simulink model "droop_model"  (R2023a)
settings: Solver=VariableStepAuto  StartTime=0.0  StopTime=6  RelTol=1e-3
values from neighbouring files (symbols this model uses):
  BESS2 =     [state_space.mat]    (also in state_space_and_controllers.mat)
  Grid =     [state_space.mat]    (also in state_space_and_controllers.mat)
  Load =     [state_space.mat]    (also in state_space_and_controllers.mat)
  PV1 =     [state_space.mat]    (also in state_space_and_controllers.mat)
  Ts = 0.0001    [cost_analysis.m]    (also in simulation_run.m)
undefined symbols (not defined in the file or in its folder): A1, A2, B1, B2, C1, C2, K1_integral, K1_proportional, K2_integral, K2_proportional
libraries: slpidlib x5, spspowerguiLib x1
settings Model: Creator=paul  LastModifiedBy=paul
settings DataIOCC: Refine=4

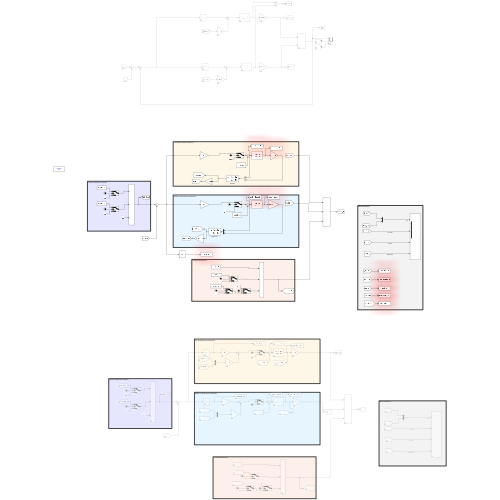
[thumbnail: Simulink's stored preview of the top-level diagram]
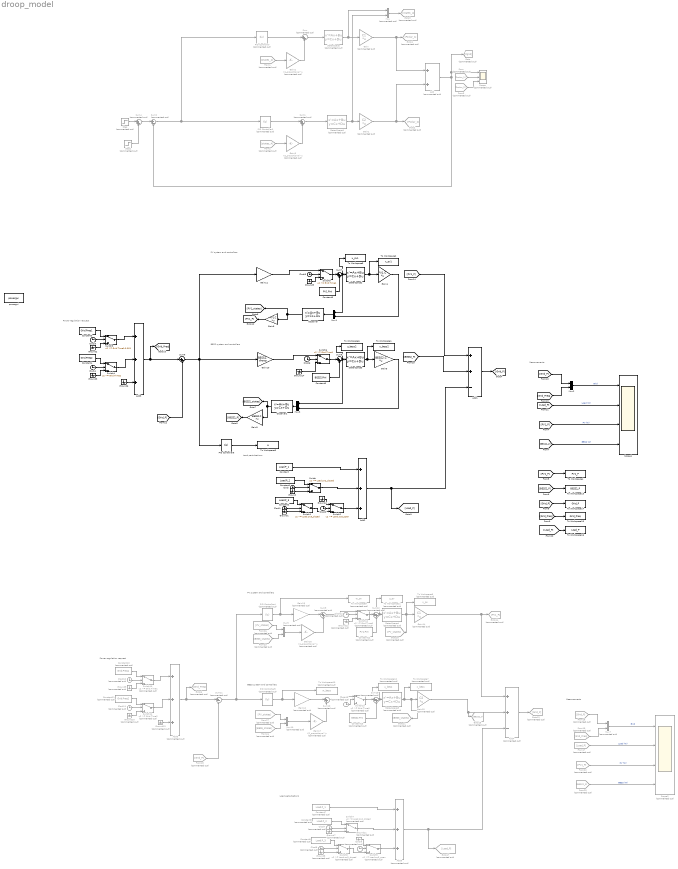
== system droop_model ==
  note: BESS system and controllers
  note: Measurements
  note: PV system and controllers
  note: Load perturbations
  note: Power regulation request
  note: BESS system and controllers
  note: Load perturbations
  note: Measurements
  note: Power regulation request
  note: PV system and controllers
  Add : Sum  Commented=on
  Add1 : Sum  Inputs=++-
  Add2 : Sum  Inputs=+++
  Add3 : Sum  Inputs=+++
  Add4 : Sum  Commented=on  Inputs=++-
  Add5 : Sum  Commented=on  Inputs=+++
  Add6 : Sum  Commented=on  Inputs=+++
  Clock{,1..6} (7 alike) : Clock
  Clock{7..13} (7 alike) : Clock  Commented=on
  Constant : Constant  Value=Load.P_1
  Constant1 : Constant  Value=Load.P_2
  Constant10 : Constant  Commented=on  Value=Grid.Preq1
  Constant11 : Constant  Commented=on  Value=Grid.Preq2
  Constant12 : Constant  Commented=on  Value=PV1.Pini
  Constant13 : Constant  Commented=on  Value=BESS2.Pini
  Constant2 : Constant  Value=Load.P_3
  Constant3 : Constant  Value=Grid.Preq1
  Constant4 : Constant  Value=Grid.Preq2
  Constant5 : Constant  Value=PV1.Pini
  Constant6 : Constant  Value=BESS2.Pini
  Constant7 : Constant  Commented=on  Value=Load.P_1
  Constant8 : Constant  Commented=on  Value=Load.P_2
  Constant9 : Constant  Commented=on  Value=Load.P_3
  From : From  Commented=on  GotoTag=Psolar_1
  From1 : From  Commented=on  GotoTag=states_4
  From16 : From  Commented=on  GotoTag=Grid_P
  From17 : From  Commented=on  GotoTag=Load_P
  From18 : From  Commented=on  GotoTag=Grid_P
  From19 : From  Commented=on  GotoTag=Grid_Preq
  From2 : From  Commented=on  GotoTag=states_4
  From22 : From  Commented=on  GotoTag=PV1_P
  From23 : From  Commented=on  GotoTag=BESS_states
  From24 : From  Commented=on  GotoTag=BESS_states
  From25 : From  Commented=on  GotoTag=BESS2_P
  From26 : From  Commented=on  GotoTag=PV_states
  From27 : From  Commented=on  GotoTag=PV_states
  From3 : From  Commented=on  GotoTag=Psolar_2
  Gain : Gain  Commented=on  Gain=C1  Multiplication=Matrix(K*u)
  Gain1 : Gain  Commented=on  Gain=C2  Multiplication=Matrix(K*u)
  Gain10 : Gain  Gain=BESS2. droop
  Gain11 : Gain  Gain=PV1.droop
  Gain12 : Gain  Commented=on  Gain=K2_integral
  Gain13 : Gain  Commented=on  Gain=K1_integral
  Gain14 : Gain  Commented=on  Gain=C1  Multiplication=Matrix(K*u)
  Gain15 : Gain  Commented=on  Gain=C2  Multiplication=Matrix(K*u)
  Gain16 : Gain  Commented=on  Gain=K1_proportional  Multiplication=Matrix(K*u)
  Gain17 : Gain  Commented=on  Gain=K2_proportional  Multiplication=Matrix(K*u)
  Gain2 : Gain  Commented=on  Gain=K1_proportional  Multiplication=Matrix(K*u)
  Gain3 : Gain  Commented=on  Gain=K2_proportional  Multiplication=Matrix(K*u)
  Gain4 : Gain  Gain=PV1.C  Multiplication=Matrix(K*u)
  Gain5 : Gain  Gain=BESS2.C  Multiplication=Matrix(K*u)
  Gain8 : Gain  Gain=PV1.C  Multiplication=Matrix(K*u)
  Gain9 : Gain  Gain=BESS2.C  Multiplication=Matrix(K*u)
  Goto : Goto  Commented=on  GotoTag=Pgrid
  Goto1 : Goto  Commented=on  GotoTag=Psolar_1
  Goto11 : Goto  Commented=on  GotoTag=BESS_states
  Goto13 : Goto  Commented=on  GotoTag=Grid_P
  Goto14 : Goto  Commented=on  GotoTag=PV1_P
  Goto15 : Goto  Commented=on  GotoTag=BESS2_P
  Goto17 : Goto  Commented=on  GotoTag=Load_P
  Goto18 : Goto  Commented=on  GotoTag=PV_states
  Goto2 : Goto  Commented=on  GotoTag=Psolar_2
  Goto3 : Goto  Commented=on  GotoTag=states_4
  Goto6 : Goto  Commented=on  GotoTag=Grid_Preq
  Ground{,1..6,14} (8 alike) : Ground
  Ground{7..13} (7 alike) : Ground  Commented=on
  Mux{,7,9..10} (4 alike) : Mux  Commented=on  Inputs=2
  Mux1 : Mux  Inputs=2
  Mux2 : Mux  Inputs=2
  Mux3 : Mux  Inputs=2
  Observer : StateSpace  A=PV1.kf_As  B=PV1.kf_Bs  C=PV1.kf_Cs  D=PV1.kf_Ds  InitialCondition=0
  Observer1 : StateSpace  A=BESS2.kf_As  B=BESS2.kf_Bs  C=BESS2.kf_Cs  D=BESS2.kf_Ds  InitialCondition=0
  PID Controller : slpidlib/PID Controller  Commented=on  Controller=I  Form=Parallel  TimeDomain=Continuous-time  UseExternalTs=off  SampleTime=-1  IntegratorMethod=Forward Euler  FilterMethod=Forward Euler  ControllerParametersSource=internal  P=1  I=K1_integral  UseKiTs=off  D=0  N=100  UseFilter=on  TunerSelectOption=Transfer Function Based (PID Tuner App)  InitialConditionSource=internal  InitialConditionForIntegrator=0  InitialConditionForFilter=0  DifferentiatorICPrevScaledInput=0  ExternalReset=none  TrackingMode=off  Kt=1  LimitOutput=off  SatLimitsSource=internal  UpperSaturationLimit=inf  LowerSaturationLimit=-inf  LinearizeAsGain=on  AntiWindupMode=none  Kb=1  LimitIntegrator=off  UpperIntegratorSaturationLimit=inf  LowerIntegratorSaturationLimit=-inf  POutMin=[]  POutMax=[]  IOutMin=[]  IOutMax=[]  DOutMin=[]  DOutMax=[]  NOutMin=[]  NOutMax=[]  SumOutMin=[]  SumOutMax=[]  SaturationOutMin=[]  SaturationOutMax=[]  PParamMin=[]  PParamMax=[]  IParamMin=[]  IParamMax=[]  DParamMin=[]  DParamMax=[]  NParamMin=[]  NParamMax=[]  KbParamMin=[]  KbParamMax=[]  KtParamMin=[]  KtParamMax=[]  KbOutMin=[]  KbOutMax=[]  KtOutMin=[]  KtOutMax=[]  IntegratorOutMin=[]  IntegratorOutMax=[]  FilterOutMin=[]  FilterOutMax=[]  SumI1OutMin=[]  SumI1OutMax=[]  SumI2OutMin=[]  SumI2OutMax=[]  SumI3OutMin=[]  SumI3OutMax=[]  SumI4OutMin=[]  SumI4OutMax=[]  SumDOutMin=[]  SumDOutMax=[]  DifferentiatorOutMin=[]  DifferentiatorOutMax=[]  FilterDiffOutCoefMin=[]  FilterDiffOutCoefMax=[]  ReciprocalOutMin=[]  ReciprocalOutMax=[]  SumDenOutMin=[]  SumDenOutMax=[]  SumNumOutMin=[]  SumNumOutMax=[]  DivideOutMin=[]  DivideOutMax=[]  UdiffTsProdOutMin=[]  UdiffTsProdOutMax=[]  NTsProdOutMin=[]  NTsProdOutMax=[]  UintegralTsProdOutMin=[]  UintegralTsProdOutMax=[]  UngainTsProdOutMin=[]  UngainTsProdOutMax=[]  ClampingZeroOutDataTypeStr=Inherit: Inherit via back propagation  ClampingZeroOutMin=[]  ClampingZeroOutMax=[]  FilterDenConstantOutDataTypeStr=Inherit: Inherit via back propagation  FilterDenConstantOutMin=[]  FilterDenConstantOutMax=[]  PCopyOutDataTypeStr=Inherit: Inherit via back propagation  PCopyOutMin=[]  PCopyOutMax=[]  NCopyOutDataTypeStr=Inherit: Inherit via back propagation  NCopyOutMin=[]  NCopyOutMax=[]  IntegratorContinuousStateAttributes=''  IntegratorStateMustResolveToSignalObject=off  IntegratorRTWStateStorageClass=Auto  FilterContinuousStateAttributes=''  FilterStateMustResolveToSignalObject=off  FilterRTWStateStorageClass=Auto  ParallelPVariant=Disabled  IdealPVariant=Disabled  IVariant=InternalParameters  DVariant=Disabled  IntegratorVariant=Continuous  SatVariant=Disabled  AWVariant=Passthrough  PCopyVariant=Disabled  TRVariant=Disabled  FdbkBlocksVariant=Forward  IdealPFdbkVariant=Disabled  SatFdbkVariant=Disabled  DerivativeFilterVariant=Disabled  NVariant=Disabled  NCopyVariant=Disabled_SignalSpec  FilterICVariant=Disabled  IntegratorICVariant=InternalICs  ExternalResetVariant=Disabled  TRSumVariant=Passthrough  SumFdbkVariant=Disabled  SumVariant=Passthrough_I  TsampFilterVariant=InternalTs  TsampNgainVariant=Passthrough  TsampIntegralVariant=Disabled_SignalSpec  ExternalSaturationOutDataTypeStr=Inherit: Same as second input
  PID Controller1 : slpidlib/PID Controller  Commented=on  Controller=I  Form=Parallel  TimeDomain=Continuous-time  UseExternalTs=off  SampleTime=-1  IntegratorMethod=Forward Euler  FilterMethod=Forward Euler  ControllerParametersSource=internal  P=1  I=K2_integral  UseKiTs=off  D=0  N=100  UseFilter=on  TunerSelectOption=Transfer Function Based (PID Tuner App)  InitialConditionSource=internal  InitialConditionForIntegrator=0  InitialConditionForFilter=0  DifferentiatorICPrevScaledInput=0  ExternalReset=none  TrackingMode=off  Kt=1  LimitOutput=off  SatLimitsSource=internal  UpperSaturationLimit=inf  LowerSaturationLimit=-inf  LinearizeAsGain=on  AntiWindupMode=none  Kb=1  LimitIntegrator=off  UpperIntegratorSaturationLimit=inf  LowerIntegratorSaturationLimit=-inf  POutMin=[]  POutMax=[]  IOutMin=[]  IOutMax=[]  DOutMin=[]  DOutMax=[]  NOutMin=[]  NOutMax=[]  SumOutMin=[]  SumOutMax=[]  SaturationOutMin=[]  SaturationOutMax=[]  PParamMin=[]  PParamMax=[]  IParamMin=[]  IParamMax=[]  DParamMin=[]  DParamMax=[]  NParamMin=[]  NParamMax=[]  KbParamMin=[]  KbParamMax=[]  KtParamMin=[]  KtParamMax=[]  KbOutMin=[]  KbOutMax=[]  KtOutMin=[]  KtOutMax=[]  IntegratorOutMin=[]  IntegratorOutMax=[]  FilterOutMin=[]  FilterOutMax=[]  SumI1OutMin=[]  SumI1OutMax=[]  SumI2OutMin=[]  SumI2OutMax=[]  SumI3OutMin=[]  SumI3OutMax=[]  SumI4OutMin=[]  SumI4OutMax=[]  SumDOutMin=[]  SumDOutMax=[]  DifferentiatorOutMin=[]  DifferentiatorOutMax=[]  FilterDiffOutCoefMin=[]  FilterDiffOutCoefMax=[]  ReciprocalOutMin=[]  ReciprocalOutMax=[]  SumDenOutMin=[]  SumDenOutMax=[]  SumNumOutMin=[]  SumNumOutMax=[]  DivideOutMin=[]  DivideOutMax=[]  UdiffTsProdOutMin=[]  UdiffTsProdOutMax=[]  NTsProdOutMin=[]  NTsProdOutMax=[]  UintegralTsProdOutMin=[]  UintegralTsProdOutMax=[]  UngainTsProdOutMin=[]  UngainTsProdOutMax=[]  ClampingZeroOutDataTypeStr=Inherit: Inherit via back propagation  ClampingZeroOutMin=[]  ClampingZeroOutMax=[]  FilterDenConstantOutDataTypeStr=Inherit: Inherit via back propagation  FilterDenConstantOutMin=[]  FilterDenConstantOutMax=[]  PCopyOutDataTypeStr=Inherit: Inherit via back propagation  PCopyOutMin=[]  PCopyOutMax=[]  NCopyOutDataTypeStr=Inherit: Inherit via back propagation  NCopyOutMin=[]  NCopyOutMax=[]  IntegratorContinuousStateAttributes=''  IntegratorStateMustResolveToSignalObject=off  IntegratorRTWStateStorageClass=Auto  FilterContinuousStateAttributes=''  FilterStateMustResolveToSignalObject=off  FilterRTWStateStorageClass=Auto  ParallelPVariant=Disabled  IdealPVariant=Disabled  IVariant=InternalParameters  DVariant=Disabled  IntegratorVariant=Continuous  SatVariant=Disabled  AWVariant=Passthrough  PCopyVariant=Disabled  TRVariant=Disabled  FdbkBlocksVariant=Forward  IdealPFdbkVariant=Disabled  SatFdbkVariant=Disabled  DerivativeFilterVariant=Disabled  NVariant=Disabled  NCopyVariant=Disabled_SignalSpec  FilterICVariant=Disabled  IntegratorICVariant=InternalICs  ExternalResetVariant=Disabled  TRSumVariant=Passthrough  SumFdbkVariant=Disabled  SumVariant=Passthrough_I  TsampFilterVariant=InternalTs  TsampNgainVariant=Passthrough  TsampIntegralVariant=Disabled_SignalSpec  ExternalSaturationOutDataTypeStr=Inherit: Same as second input
  PID Controller4 : slpidlib/PID Controller  Commented=on  Controller=I  Form=Parallel  TimeDomain=Continuous-time  UseExternalTs=off  SampleTime=-1  IntegratorMethod=Forward Euler  FilterMethod=Forward Euler  ControllerParametersSource=internal  P=1  I=1  UseKiTs=off  D=0  N=100  UseFilter=on  TunerSelectOption=Transfer Function Based (PID Tuner App)  InitialConditionSource=internal  InitialConditionForIntegrator=0  InitialConditionForFilter=0  DifferentiatorICPrevScaledInput=0  ExternalReset=none  TrackingMode=off  Kt=1  LimitOutput=off  SatLimitsSource=internal  UpperSaturationLimit=inf  LowerSaturationLimit=-inf  LinearizeAsGain=on  AntiWindupMode=none  Kb=1  LimitIntegrator=off  UpperIntegratorSaturationLimit=inf  LowerIntegratorSaturationLimit=-inf  POutMin=[]  POutMax=[]  IOutMin=[]  IOutMax=[]  DOutMin=[]  DOutMax=[]  NOutMin=[]  NOutMax=[]  SumOutMin=[]  SumOutMax=[]  SaturationOutMin=[]  SaturationOutMax=[]  PParamMin=[]  PParamMax=[]  IParamMin=[]  IParamMax=[]  DParamMin=[]  DParamMax=[]  NParamMin=[]  NParamMax=[]  KbParamMin=[]  KbParamMax=[]  KtParamMin=[]  KtParamMax=[]  KbOutMin=[]  KbOutMax=[]  KtOutMin=[]  KtOutMax=[]  IntegratorOutMin=[]  IntegratorOutMax=[]  FilterOutMin=[]  FilterOutMax=[]  SumI1OutMin=[]  SumI1OutMax=[]  SumI2OutMin=[]  SumI2OutMax=[]  SumI3OutMin=[]  SumI3OutMax=[]  SumI4OutMin=[]  SumI4OutMax=[]  SumDOutMin=[]  SumDOutMax=[]  DifferentiatorOutMin=[]  DifferentiatorOutMax=[]  FilterDiffOutCoefMin=[]  FilterDiffOutCoefMax=[]  ReciprocalOutMin=[]  ReciprocalOutMax=[]  SumDenOutMin=[]  SumDenOutMax=[]  SumNumOutMin=[]  SumNumOutMax=[]  DivideOutMin=[]  DivideOutMax=[]  UdiffTsProdOutMin=[]  UdiffTsProdOutMax=[]  NTsProdOutMin=[]  NTsProdOutMax=[]  UintegralTsProdOutMin=[]  UintegralTsProdOutMax=[]  UngainTsProdOutMin=[]  UngainTsProdOutMax=[]  ClampingZeroOutDataTypeStr=Inherit: Inherit via back propagation  ClampingZeroOutMin=[]  ClampingZeroOutMax=[]  FilterDenConstantOutDataTypeStr=Inherit: Inherit via back propagation  FilterDenConstantOutMin=[]  FilterDenConstantOutMax=[]  PCopyOutDataTypeStr=Inherit: Inherit via back propagation  PCopyOutMin=[]  PCopyOutMax=[]  NCopyOutDataTypeStr=Inherit: Inherit via back propagation  NCopyOutMin=[]  NCopyOutMax=[]  IntegratorContinuousStateAttributes=''  IntegratorStateMustResolveToSignalObject=off  IntegratorRTWStateStorageClass=Auto  FilterContinuousStateAttributes=''  FilterStateMustResolveToSignalObject=off  FilterRTWStateStorageClass=Auto  ParallelPVariant=Disabled  IdealPVariant=Disabled  IVariant=InternalParameters  DVariant=Disabled  IntegratorVariant=Continuous  SatVariant=Disabled  AWVariant=Passthrough  PCopyVariant=Disabled  TRVariant=Disabled  FdbkBlocksVariant=Forward  IdealPFdbkVariant=Disabled  SatFdbkVariant=Disabled  DerivativeFilterVariant=Disabled  NVariant=Disabled  NCopyVariant=Disabled_SignalSpec  FilterICVariant=Disabled  IntegratorICVariant=InternalICs  ExternalResetVariant=Disabled  TRSumVariant=Passthrough  SumFdbkVariant=Disabled  SumVariant=Passthrough_I  TsampFilterVariant=InternalTs  TsampNgainVariant=Passthrough  TsampIntegralVariant=Disabled_SignalSpec  ExternalSaturationOutDataTypeStr=Inherit: Same as second input
  PID Controller5 : slpidlib/PID Controller  Commented=on  Controller=I  Form=Parallel  TimeDomain=Continuous-time  UseExternalTs=off  SampleTime=-1  IntegratorMethod=Forward Euler  FilterMethod=Forward Euler  ControllerParametersSource=internal  P=1  I=1  UseKiTs=off  D=0  N=100  UseFilter=on  TunerSelectOption=Transfer Function Based (PID Tuner App)  InitialConditionSource=internal  InitialConditionForIntegrator=0  InitialConditionForFilter=0  DifferentiatorICPrevScaledInput=0  ExternalReset=none  TrackingMode=off  Kt=1  LimitOutput=off  SatLimitsSource=internal  UpperSaturationLimit=inf  LowerSaturationLimit=-inf  LinearizeAsGain=on  AntiWindupMode=none  Kb=1  LimitIntegrator=off  UpperIntegratorSaturationLimit=inf  LowerIntegratorSaturationLimit=-inf  POutMin=[]  POutMax=[]  IOutMin=[]  IOutMax=[]  DOutMin=[]  DOutMax=[]  NOutMin=[]  NOutMax=[]  SumOutMin=[]  SumOutMax=[]  SaturationOutMin=[]  SaturationOutMax=[]  PParamMin=[]  PParamMax=[]  IParamMin=[]  IParamMax=[]  DParamMin=[]  DParamMax=[]  NParamMin=[]  NParamMax=[]  KbParamMin=[]  KbParamMax=[]  KtParamMin=[]  KtParamMax=[]  KbOutMin=[]  KbOutMax=[]  KtOutMin=[]  KtOutMax=[]  IntegratorOutMin=[]  IntegratorOutMax=[]  FilterOutMin=[]  FilterOutMax=[]  SumI1OutMin=[]  SumI1OutMax=[]  SumI2OutMin=[]  SumI2OutMax=[]  SumI3OutMin=[]  SumI3OutMax=[]  SumI4OutMin=[]  SumI4OutMax=[]  SumDOutMin=[]  SumDOutMax=[]  DifferentiatorOutMin=[]  DifferentiatorOutMax=[]  FilterDiffOutCoefMin=[]  FilterDiffOutCoefMax=[]  ReciprocalOutMin=[]  ReciprocalOutMax=[]  SumDenOutMin=[]  SumDenOutMax=[]  SumNumOutMin=[]  SumNumOutMax=[]  DivideOutMin=[]  DivideOutMax=[]  UdiffTsProdOutMin=[]  UdiffTsProdOutMax=[]  NTsProdOutMin=[]  NTsProdOutMax=[]  UintegralTsProdOutMin=[]  UintegralTsProdOutMax=[]  UngainTsProdOutMin=[]  UngainTsProdOutMax=[]  ClampingZeroOutDataTypeStr=Inherit: Inherit via back propagation  ClampingZeroOutMin=[]  ClampingZeroOutMax=[]  FilterDenConstantOutDataTypeStr=Inherit: Inherit via back propagation  FilterDenConstantOutMin=[]  FilterDenConstantOutMax=[]  PCopyOutDataTypeStr=Inherit: Inherit via back propagation  PCopyOutMin=[]  PCopyOutMax=[]  NCopyOutDataTypeStr=Inherit: Inherit via back propagation  NCopyOutMin=[]  NCopyOutMax=[]  IntegratorContinuousStateAttributes=''  IntegratorStateMustResolveToSignalObject=off  IntegratorRTWStateStorageClass=Auto  FilterContinuousStateAttributes=''  FilterStateMustResolveToSignalObject=off  FilterRTWStateStorageClass=Auto  ParallelPVariant=Disabled  IdealPVariant=Disabled  IVariant=InternalParameters  DVariant=Disabled  IntegratorVariant=Continuous  SatVariant=Disabled  AWVariant=Passthrough  PCopyVariant=Disabled  TRVariant=Disabled  FdbkBlocksVariant=Forward  IdealPFdbkVariant=Disabled  SatFdbkVariant=Disabled  DerivativeFilterVariant=Disabled  NVariant=Disabled  NCopyVariant=Disabled_SignalSpec  FilterICVariant=Disabled  IntegratorICVariant=InternalICs  ExternalResetVariant=Disabled  TRSumVariant=Passthrough  SumFdbkVariant=Disabled  SumVariant=Passthrough_I  TsampFilterVariant=InternalTs  TsampNgainVariant=Passthrough  TsampIntegralVariant=Disabled_SignalSpec  ExternalSaturationOutDataTypeStr=Inherit: Same as second input
  PID Controller6 : slpidlib/PID Controller  Controller=I  Form=Parallel  TimeDomain=Continuous-time  UseExternalTs=off  SampleTime=-1  IntegratorMethod=Forward Euler  FilterMethod=Forward Euler  ControllerParametersSource=internal  P=1  I=1  UseKiTs=off  D=0  N=100  UseFilter=on  TunerSelectOption=Transfer Function Based (PID Tuner App)  InitialConditionSource=internal  InitialConditionForIntegrator=0  InitialConditionForFilter=0  DifferentiatorICPrevScaledInput=0  ExternalReset=none  TrackingMode=off  Kt=1  LimitOutput=off  SatLimitsSource=internal  UpperSaturationLimit=inf  LowerSaturationLimit=-inf  LinearizeAsGain=on  AntiWindupMode=none  Kb=1  LimitIntegrator=off  UpperIntegratorSaturationLimit=inf  LowerIntegratorSaturationLimit=-inf  POutMin=[]  POutMax=[]  IOutMin=[]  IOutMax=[]  DOutMin=[]  DOutMax=[]  NOutMin=[]  NOutMax=[]  SumOutMin=[]  SumOutMax=[]  SaturationOutMin=[]  SaturationOutMax=[]  PParamMin=[]  PParamMax=[]  IParamMin=[]  IParamMax=[]  DParamMin=[]  DParamMax=[]  NParamMin=[]  NParamMax=[]  KbParamMin=[]  KbParamMax=[]  KtParamMin=[]  KtParamMax=[]  KbOutMin=[]  KbOutMax=[]  KtOutMin=[]  KtOutMax=[]  IntegratorOutMin=[]  IntegratorOutMax=[]  FilterOutMin=[]  FilterOutMax=[]  SumI1OutMin=[]  SumI1OutMax=[]  SumI2OutMin=[]  SumI2OutMax=[]  SumI3OutMin=[]  SumI3OutMax=[]  SumI4OutMin=[]  SumI4OutMax=[]  SumDOutMin=[]  SumDOutMax=[]  DifferentiatorOutMin=[]  DifferentiatorOutMax=[]  FilterDiffOutCoefMin=[]  FilterDiffOutCoefMax=[]  ReciprocalOutMin=[]  ReciprocalOutMax=[]  SumDenOutMin=[]  SumDenOutMax=[]  SumNumOutMin=[]  SumNumOutMax=[]  DivideOutMin=[]  DivideOutMax=[]  UdiffTsProdOutMin=[]  UdiffTsProdOutMax=[]  NTsProdOutMin=[]  NTsProdOutMax=[]  UintegralTsProdOutMin=[]  UintegralTsProdOutMax=[]  UngainTsProdOutMin=[]  UngainTsProdOutMax=[]  ClampingZeroOutDataTypeStr=Inherit: Inherit via back propagation  ClampingZeroOutMin=[]  ClampingZeroOutMax=[]  FilterDenConstantOutDataTypeStr=Inherit: Inherit via back propagation  FilterDenConstantOutMin=[]  FilterDenConstantOutMax=[]  PCopyOutDataTypeStr=Inherit: Inherit via back propagation  PCopyOutMin=[]  PCopyOutMax=[]  NCopyOutDataTypeStr=Inherit: Inherit via back propagation  NCopyOutMin=[]  NCopyOutMax=[]  IntegratorContinuousStateAttributes=''  IntegratorStateMustResolveToSignalObject=off  IntegratorRTWStateStorageClass=Auto  FilterContinuousStateAttributes=''  FilterStateMustResolveToSignalObject=off  FilterRTWStateStorageClass=Auto  ParallelPVariant=Disabled  IdealPVariant=Disabled  IVariant=InternalParameters  DVariant=Disabled  IntegratorVariant=Continuous  SatVariant=Disabled  AWVariant=Passthrough  PCopyVariant=Disabled  TRVariant=Disabled  FdbkBlocksVariant=Forward  IdealPFdbkVariant=Disabled  SatFdbkVariant=Disabled  DerivativeFilterVariant=Disabled  NVariant=Disabled  NCopyVariant=Disabled_SignalSpec  FilterICVariant=Disabled  IntegratorICVariant=InternalICs  ExternalResetVariant=Disabled  TRSumVariant=Passthrough  SumFdbkVariant=Disabled  SumVariant=Passthrough_I  TsampFilterVariant=InternalTs  TsampNgainVariant=Passthrough  TsampIntegralVariant=Disabled_SignalSpec  ExternalSaturationOutDataTypeStr=Inherit: Same as second input
  Scope : Scope  Commented=on  NumInputPorts=3
  Scope1 : Scope  NumInputPorts=4
  Scope2 : Scope  Commented=on  NumInputPorts=4
  State-Space : StateSpace  Commented=on  A=A1  B=[1; 0]  C=[1 0;0 1]  D=zeros(2,1)  InitialCondition=0
  State-Space1 : StateSpace  Commented=on  A=A2  B=[1; 0]  C=[1 0;0 1]  D=zeros(2,1)  InitialCondition=0
  State-Space2 : StateSpace  A=PV1.A  B=PV1.B  C=eye(2,2)  D=zeros(2,1)  InitialCondition=0
  State-Space3 : StateSpace  A=BESS2.A  B=BESS2.B  C=eye(2,2)  D=zeros(2,1)  InitialCondition=0
  State-Space4 : StateSpace  Commented=on  A=A1  B=B1  C=eye(2,2)  D=zeros(2,1)  InitialCondition=0
  State-Space5 : StateSpace  Commented=on  A=A2  B=B2  C=eye(2,2)  D=zeros(2,1)  InitialCondition=0
  Step : Step  Commented=on  After=1.5*10^6  SampleTime=0
  Step1 : Step  Commented=on  Time=15  After=0.5*10^6  SampleTime=0
  Sum{,1,4,9..10,12..13} (7 alike) : Sum  Commented=on  Inputs=|++
  Sum11 : Sum  Commented=on  Inputs=|+-
  Sum2 : Sum  Commented=on  Inputs=|+-
  Sum6 : Sum  Inputs=|+-
  Sum7 : Sum  Inputs=|++
  Sum8 : Sum  Inputs=|++
  Switch : Switch  Threshold=Load.sw2_closed  SaturateOnIntegerOverflow=off  InputSameDT=off
  Switch1 : Switch  Threshold=Load.sw3_closed  SaturateOnIntegerOverflow=off  InputSameDT=off
  Switch10 : Switch  Commented=on  Threshold=Grid.Time1  SaturateOnIntegerOverflow=off  InputSameDT=off
  Switch11 : Switch  Commented=on  Threshold=Grid.Time2  SaturateOnIntegerOverflow=off  InputSameDT=off
  Switch12 : Switch  Commented=on  Threshold=Grid.Time0  SaturateOnIntegerOverflow=off  InputSameDT=off
  Switch13 : Switch  Commented=on  Threshold=Grid.Time0  SaturateOnIntegerOverflow=off  InputSameDT=off
  Switch2 : Switch  Threshold=Load.sw3_open  SaturateOnIntegerOverflow=off  InputSameDT=off
  Switch3 : Switch  Threshold=Grid.Time1-0.001  SaturateOnIntegerOverflow=off  InputSameDT=off
  Switch4 : Switch  Threshold=Grid.Time2  SaturateOnIntegerOverflow=off  InputSameDT=off
  Switch5 : Switch  Threshold=Grid.Time1  SaturateOnIntegerOverflow=off  InputSameDT=off
  Switch6 : Switch  Threshold=Grid.Time1  SaturateOnIntegerOverflow=off  InputSameDT=off
  Switch7 : Switch  Commented=on  Threshold=Load.sw2_closed  SaturateOnIntegerOverflow=off  InputSameDT=off
  Switch8 : Switch  Commented=on  Threshold=Load.sw3_closed  SaturateOnIntegerOverflow=off  InputSameDT=off
  Switch9 : Switch  Commented=on  Threshold=Load.sw3_open  SaturateOnIntegerOverflow=off  InputSameDT=off
  To Workspace1 : ToWorkspace  VariableName=x_bess2  SaveFormat=Timeseries  SampleTime=Ts
  To Workspace10 : ToWorkspace  Commented=on  VariableName=w_bess  SaveFormat=Timeseries  SampleTime=Ts
  To Workspace11 : ToWorkspace  Commented=on  VariableName=u_pv  SaveFormat=Timeseries  SampleTime=Ts
  To Workspace12 : ToWorkspace  Commented=on  VariableName=u_bess  SaveFormat=Timeseries  SampleTime=Ts
  To Workspace13 : ToWorkspace  VariableName=BESS2_P  SaveFormat=Timeseries  SampleTime=Ts
  To Workspace14 : ToWorkspace  VariableName=Grid_P  SaveFormat=Timeseries  SampleTime=Ts
  To Workspace15 : ToWorkspace  VariableName=Grid_Preq  SaveFormat=Timeseries  SampleTime=Ts
  To Workspace16 : ToWorkspace  VariableName=Load_P  SaveFormat=Timeseries  SampleTime=Ts
  To Workspace2 : ToWorkspace  VariableName=x_pv1  SaveFormat=Timeseries  SampleTime=Ts
  To Workspace3 : ToWorkspace  VariableName=w  SaveFormat=Timeseries  SampleTime=Ts
  To Workspace4 : ToWorkspace  VariableName=PV1_P  SaveFormat=Timeseries  SampleTime=Ts
  To Workspace5 : ToWorkspace  VariableName=u_pv1  SaveFormat=Timeseries  SampleTime=Ts
  To Workspace6 : ToWorkspace  VariableName=u_bess2  SaveFormat=Timeseries  SampleTime=Ts
  To Workspace7 : ToWorkspace  Commented=on  VariableName=x_bess  SaveFormat=Timeseries  SampleTime=Ts
  To Workspace8 : ToWorkspace  Commented=on  VariableName=x_pv  SaveFormat=Timeseries  SampleTime=Ts
  To Workspace9 : ToWorkspace  Commented=on  VariableName=w_pv  SaveFormat=Timeseries  SampleTime=Ts
  powergui : spspowerguiLib/powergui  Priority=1  SimulationMode=Discrete  SampleTime=Ts  frequency=60  Iterations=50  frequencyindice=60  Pbase=100e6  ErrMax=1e-4  UnitsV=kV  UnitsW=MW  buscounter=0  FunctionMessages=off  echomessages=off  EnableUseOfTLC=off  CurrentSourceSwitches=off  DisableSnubberDevices=off  DisableRonSwitches=off  DisableVfSwitches=off  DisplayEquations=off  AutomaticDiscreteSolvers=off  SolverType=Tustin/Backward Euler (TBE)  Interpol=off  ExternalGateDelay=off  methode=off  Ts=100  x0status=blocks  SPID=on  SwTol=0  HookPort=off  NonlinearTolerance=1e-4  nMaxIteration=100  ContinueOnMaxIteration=off  RestoreLinks=warning  ResistiveCurrentMeasurement=off  Frange=[0:2:500]  Ylog=off  Xlog=on  ShowGrid=off  save=off  variable=ZData  structure=0  ZoomFFT=off  StartTime=0.0  cycles=1  DisplayStyle=1  fundamental=60  FreqAxis=off  MaxFrequency=1000  frequencyindicesteady=1  RmsSteady=1  display=off
  wires:
  Gain/1 -> Goto1/1, Add/1
  State-Space1/1 -> Mux/2, Gain1/1
  Add/1 -> Scope/1, Goto/1, Sum2/2
  Sum/1 -> State-Space/1
  Sum1/1 -> State-Space1/1
  PID Controller1/1 -> Sum1/1
  PID Controller/1 -> Sum/1
  Sum2/1 -> PID Controller/1, PID Controller1/1
  From/1 -> Scope/2
  From3/1 -> Scope/3
  State-Space/1 -> Mux/1, Gain/1
  Gain1/1 -> Goto2/1, Add/2
  Mux/1 -> Goto3/1
  From1/1 -> Gain2/1
  Gain2/1 -> Sum/2
  From2/1 -> Gain3/1
  Gain3/1 -> Sum1/2
  Step/1 -> Sum4/1
  Sum4/1 -> Sum2/1
  Step1/1 -> Sum4/2
  Mux1/1 -> Observer/1
  Add1/1 -> [Grid_P]
  [BESS2_P] -> Scope1/4  "BESS (W)"
  Gain11/1 -> Switch5/1
  State-Space2/1 -> To Workspace2/1, Gain4/1
  State-Space3/1 -> To Workspace1/1, Gain5/1
  Sum6/1 -> PID Controller6/1, Gain11/1, Gain10/1
  [PV1_P] -> Scope1/3  "PV (W)"
  Gain5/1 -> Mux3/2
  Mux3/1 -> Observer1/1
  Gain10/1 -> Switch6/1
  Observer/1 -> Gain8/1, [PV1_states]
  Observer1/1 -> Gain9/1, [BESS2_states]
  Constant/1 -> Add2/1
  Constant1/1 -> Switch/1
  Clock/1 -> Switch/2
  Ground/1 -> Switch/3
  Switch/1 -> Add2/2
  [Load_P] -> Scope1/2  "Load (W)"
  [Grid_P] -> Sum6/2
  Ground1/1 -> Switch1/3
  Constant2/1 -> Switch1/1
  Clock1/1 -> Switch1/2
  Switch2/1 -> Add2/3
  Clock2/1 -> Switch2/2
  Switch1/1 -> Switch2/3
  Constant3/1 -> Switch3/1
  Clock3/1 -> Switch3/2
  Ground2/1 -> Switch3/3
  Switch3/1 -> Add3/1
  Add3/1 -> [Grid_Preq], Sum6/1
  Clock4/1 -> Switch4/2
  Constant4/1 -> Switch4/1
  Ground3/1 -> Switch4/3
  Switch4/1 -> Add3/2
  [Grid_P] -> Mux2/1
  Mux2/1 -> Scope1/1  "Grid"
  [Grid_Preq] -> Mux2/2
  Ground4/1 -> Switch2/1
  Constant5/1 -> Sum7/2
  Sum7/1 -> To Workspace5/1, Mux1/1, State-Space2/1
  Constant6/1 -> Sum8/2
  Sum8/1 -> Mux3/1, To Workspace6/1, State-Space3/1
  Switch5/1 -> Sum7/1
  Clock5/1 -> Switch5/2
  Switch6/1 -> Sum8/1
  Clock6/1 -> Switch6/2
  Ground5/1 -> Switch5/3
  Ground6/1 -> Add3/3
  Gain4/1 -> Mux1/2
  Add2/1 -> [Load_P], Add1/3
  Gain8/1 -> [PV1_P]
  [PV1_P] -> Add1/1
  Gain9/1 -> [BESS2_P]
  Ground8/1 -> Switch8/3
  Ground7/1 -> Switch7/3
  Clock13/1 -> Switch13/2
  Clock8/1 -> Switch8/2
  Switch11/1 -> Add6/2
  Ground11/1 -> Switch9/1
  State-Space4/1 -> To Workspace8/1, Goto18/1, Gain14/1
  Mux9/1 -> Gain16/1
  From27/1 -> Mux10/1
  Mux10/1 -> Gain17/1
  Sum12/1 -> To Workspace11/1, State-Space4/1
  Sum11/1 -> PID Controller4/1, PID Controller5/1
  From16/1 -> Mux7/1
  From24/1 -> Mux10/2
  PID Controller5/1 -> To Workspace10/1, Gain12/1
  Clock9/1 -> Switch9/2
  Ground13/1 -> Add6/3
  Constant12/1 -> Sum12/2
  Add5/1 -> Goto17/1, Add4/3
  Constant13/1 -> Sum13/2
  Add6/1 -> Goto6/1, Sum11/1
  Clock10/1 -> Switch10/2
  Clock12/1 -> Switch12/2
  Switch13/1 -> Sum13/1
  Sum10/1 -> Switch13/1
  Gain16/1 -> Sum9/2
  Gain17/1 -> Sum10/2
  From23/1 -> Mux9/2
  Gain12/1 -> Sum10/1
  State-Space5/1 -> To Workspace7/1, Goto11/1, Gain15/1
  Constant8/1 -> Switch7/1
  Switch7/1 -> Add5/2
  Constant7/1 -> Add5/1
  Gain15/1 -> Goto15/1, Add4/2
  Switch8/1 -> Switch9/3
  Ground12/1 -> Switch12/3
  Gain13/1 -> Sum9/1
  Gain14/1 -> Goto14/1, Add4/1
  PID Controller4/1 -> To Workspace9/1, Gain13/1
  From22/1 -> Scope2/3  "PV (W)"
  From18/1 -> Sum11/2
  Ground9/1 -> Switch10/3
  Sum9/1 -> Switch12/1
  From25/1 -> Scope2/4  "BESS (W)"
  Add4/1 -> Goto13/1
  Clock7/1 -> Switch7/2
  Constant10/1 -> Switch10/1
  Switch12/1 -> Sum12/1
  Switch9/1 -> Add5/3
  From17/1 -> Scope2/2  "Load (W)"
  Switch10/1 -> Add6/1
  Mux7/1 -> Scope2/1  "Grid"
  From26/1 -> Mux9/1
  Clock11/1 -> Switch11/2
  Constant11/1 -> Switch11/1
  Constant9/1 -> Switch8/1
  Ground10/1 -> Switch11/3
  Sum13/1 -> To Workspace12/1, State-Space5/1
  From19/1 -> Mux7/2
  Ground14/1 -> Switch6/3
  PID Controller6/1 -> To Workspace3/1
  [BESS2_P] -> Add1/2
  [BESS2_P] -> To Workspace13/1
  [PV1_P] -> To Workspace4/1
  [Grid_P] -> To Workspace14/1
  [Grid_Preq] -> To Workspace15/1
  [Load_P] -> To Workspace16/1
